simulink model "dwa"  (R2016a)
settings: Solver=VariableStepAuto  StartTime=0.0  StopTime=1  FixedStep=5e-5  RelTol=1e-3
values from neighbouring files (symbols this model uses):
  A_lpf = [-284 -370; 370 0]    [main.m]
  alpha = 0.5    [main.m]
  B_lpf = [440; 0]    [main.m]
  c = 3.5e-2    (= 0.035)    [main.m]
  C_lpf = [0 0.596]    [main.m]
  F_max = 250    [main.m]
  k = 42    [main.m]    (also in test_usw.m = [3,0.1])
  k_ac = 51    [main.m]
  k_af = 2.59e-2    (= 0.0259)    [main.m]
  L = 0.1    [main.m]
  m_c = 8.5    [main.m]
  m_f = 0.7e-3    (= 0.0007)    [main.m]
  n = 1e-18    [main.m]
  q1 = 1.53e-6    (= 1.53e-06)    [main.m]
  q2 = 0.465    [main.m]
  S = [-1.7e6 2.28e4 225 1.91 2.71]    [main.m]
  T = 0.55    [main.m]
  T_s = 5    [main.m]
undefined symbols (not defined in the file or in its folder): Discrete, sigbuilder_block, Time
libraries: simulink x1, ctrlSharedLib x1
settings Model: Creator=chao  LastModifiedBy=chao
settings GRTTargetCC: GeneratePreprocessorConditionals=Use local settings

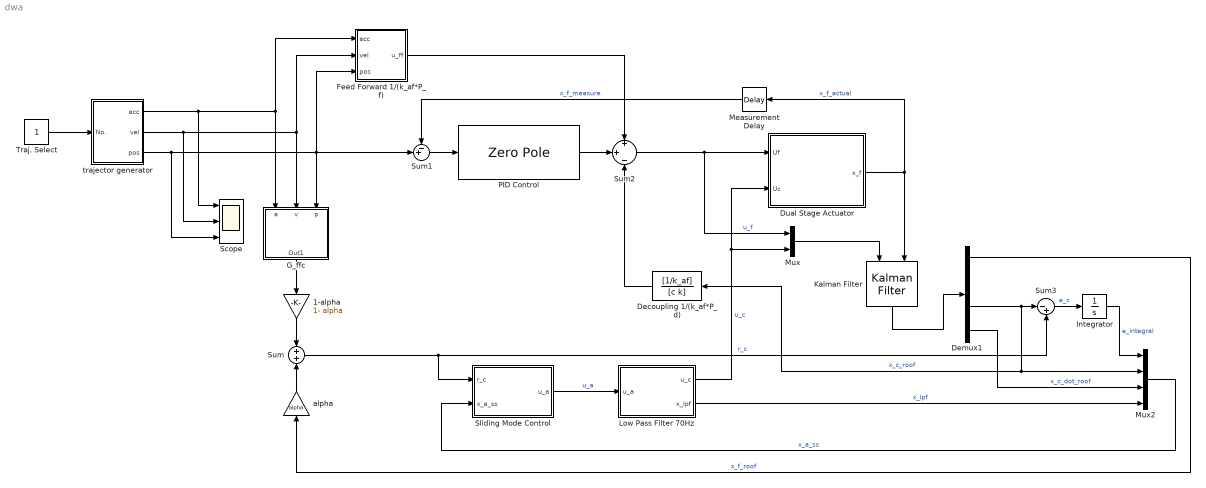
== system dwa ==
  1-alpha : Gain  Gain=1- alpha
  Decoupling 1/(k_af*P_d) : TransferFcn  Numerator=[1/k_af]  Denominator=[c k]
  Demux1 : Demux
  Dual Stage Actuator : Subsystem
  Feed Forward 1/(k_af*P_f) : Subsystem
  G_ffc : Subsystem
  Integrator : Integrator
  Kalman Filter : ctrlSharedLib/Kalman Filter  TimeDomain=Discrete-Time  UseCurrentEstimator=on  ModelSource=Individual A, B, C, D matrices  ModelSourceVariable=ss(0.95,1,1,0,1)  A=[0, 1, 0, 0; -k/m_f, -c/m_f, k/m_f, c/m_f;0, 0, 0, 1; 0, 0, 0, 0]  B=[0, 0; k_af/m_f, 0;0, 0; 0, k_ac/m_c];  C=[1 0 0 0]  D=[0 0]  NumberOfStates=1  NumberOfInputs=1  NumberOfOutputs=1  InitialEstimateSource=Dialog  X0=[0 0 0 0]  P0=10  UseK=off  UseGH=off  NumberOfProcessNoiseInputs=1  G=1  TimeInvariantG=on  H=0  TimeInvariantH=on  Q=[q1 0; 0 q2]  TimeInvariantQ=on  R=n  TimeInvariantR=on  N=0  TimeInvariantN=on  AddInputPort=on  AddEnablePort=off  OutputEstimatedY=off  OutputP=off  Ts=-1
  Low Pass Filter 70Hz : Subsystem
  Measurement Delay : TransportDelay  DelayTime=0
  Mux : Mux  Inputs=2
  Mux2 : Mux
  PID Control : ZeroPole  Zeros=[-2*pi*100 -2*pi*333]  Poles=[0 -2*pi*3000]  Gain=[3.2e6]
  Scope : Scope  NumInputPorts=3
  Sliding Mode Control : Subsystem
  Sum : Sum  Inputs=+|+
  Sum1 : Sum  Inputs=-+|
  Sum2 : Sum  Inputs=+|+|-
  Sum3 : Sum  Inputs=|-+
  Traj. Select : Constant
  alpha : Gain  Gain=alpha
  trajector generator : Subsystem
  wires:
  Sum1/1 -> PID Control/1
  PID Control/1 -> Sum2/2
  Sum2/1 -> Mux/1, Dual Stage Actuator/1(Uf)  "u_f"
  Feed Forward 1/(k_af*P_f)/1(u_ff) -> Sum2/1
  Measurement Delay/1 -> Sum1/1  "x_f_measure"
  Mux/1 -> Kalman Filter/1
  Sum3/1 -> Integrator/1  "e_c"
  Kalman Filter/1 -> Demux1/1
  Demux1/3 -> Mux2/2, Decoupling 1/(k_af*P_d)/1, Sum3/1  "x_c_roof"
  Dual Stage Actuator/1(x_f) -> Measurement Delay/1, Kalman Filter/2  "x_f_actual"
  Integrator/1 -> Mux2/1  "e_integral"
  Demux1/4 -> Mux2/3  "x_c_dot_roof"
  Low Pass Filter 70Hz/1(u_c) -> Dual Stage Actuator/2(Uc), Mux/2  "u_c"
  Mux2/1 -> Sliding Mode Control/2(x_a_ss)  "x_a_ss"
  Sliding Mode Control/1(u_a) -> Low Pass Filter 70Hz/1(u_a)  "u_a"
  Low Pass Filter 70Hz/2(x_lpf) -> Mux2/4  "x_lpf"
  Decoupling 1/(k_af*P_d)/1 -> Sum2/3
  alpha/1 -> Sum/2
  1-alpha/1 -> Sum/1
  Sum/1 -> Sliding Mode Control/1(r_c), Sum3/2  "r_c"
  Demux1/1 -> alpha/1  "x_f_roof"
  trajector generator/3(pos) -> Scope/3, Sum1/2, G_ffc/3(p), Feed Forward 1/(k_af*P_f)/3(pos)
  trajector generator/1(acc) -> Scope/1, G_ffc/1(a), Feed Forward 1/(k_af*P_f)/1(acc)
  trajector generator/2(vel) -> Scope/2, G_ffc/2(v), Feed Forward 1/(k_af*P_f)/2(vel)
  Traj. Select/1 -> trajector generator/1(No.)
  G_ffc/1(Out1) -> 1-alpha/1

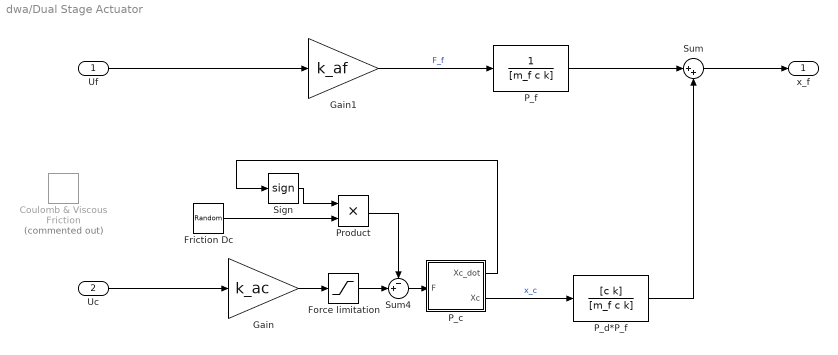
== system dwa/Dual Stage Actuator ==
  Uf : Inport
  Uc : Inport  Port=2
  Coulomb & Viscous Friction : simulink/Discontinuities/Coulomb & Viscous Friction  Commented=on  offset=[1 3 2 0]  gain=1
  Force limitation : Saturate  UpperLimit=F_max  LowerLimit=-F_max
  Friction Dc : RandomNumber  Mean=19  Variance=6.1^2  SampleTime=0.1
  Gain : Gain  Gain=k_ac
  Gain1 : Gain  Gain=k_af
  P_c : Subsystem
  P_d*P_f : TransferFcn  Numerator=[c k]  Denominator=[m_f c k]
  P_f : TransferFcn  Denominator=[m_f c k]
  Product : Product
  Sign : Signum
  Sum : Sum  Inputs=|++
  Sum4 : Sum  Inputs=-+|
  x_f : Outport
  wires:
  Gain1/1 -> P_f/1  "F_f"
  P_c/2(Xc) -> P_d*P_f/1  "x_c"
  Uf/1 -> Gain1/1
  Uc/1 -> Gain/1
  Gain/1 -> Force limitation/1
  Force limitation/1 -> Sum4/2
  Sum4/1 -> P_c/1(F)
  Friction Dc/1 -> Product/2
  Product/1 -> Sum4/1
  P_f/1 -> Sum/1
  Sum/1 -> x_f/1
  P_d*P_f/1 -> Sum/2
  P_c/1(Xc_dot) -> Sign/1
  Sign/1 -> Product/1

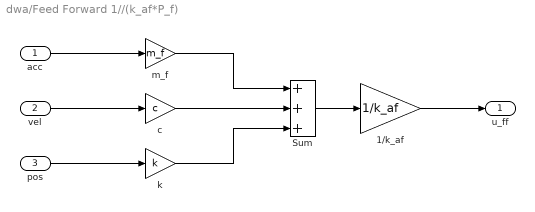
== system dwa/Feed Forward 1//(k_af*P_f) ==
  acc : Inport
  vel : Inport  Port=2
  pos : Inport  Port=3
  1/k_af : Gain  Gain=1/k_af
  Sum : Sum  Inputs=+++
  c : Gain  Gain=c
  k : Gain  Gain=k
  m_f : Gain  Gain=m_f
  u_ff : Outport
  wires:
  c/1 -> Sum/2
  acc/1 -> m_f/1
  pos/1 -> k/1
  k/1 -> Sum/3
  vel/1 -> c/1
  m_f/1 -> Sum/1
  1/k_af/1 -> u_ff/1
  Sum/1 -> 1/k_af/1

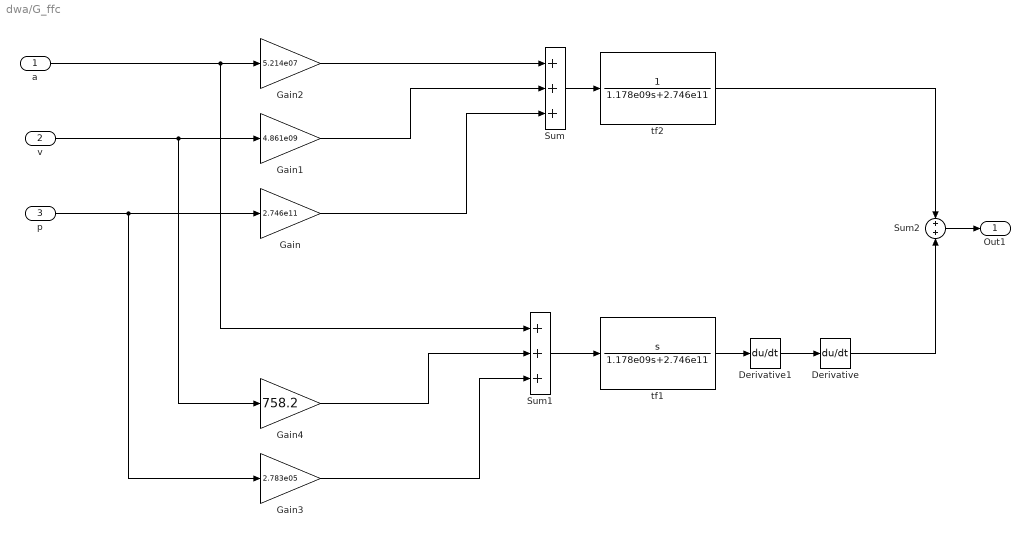
== system dwa/G_ffc ==
  a : Inport
  v : Inport  Port=2
  p : Inport  Port=3
  Derivative : Derivative
  Derivative1 : Derivative
  Gain : Gain  Gain=2.746e11
  Gain1 : Gain  Gain=4.861e09
  Gain2 : Gain  Gain=5.214e07
  Gain3 : Gain  Gain=2.783e05
  Gain4 : Gain  Gain=758.2
  Sum : Sum  Inputs=3
  Sum1 : Sum  Inputs=3
  Sum2 : Sum  Inputs=2
  tf1 : TransferFcn  Numerator="[1  0]"  Denominator=[1.178e09 2.746e11]
  tf2 : TransferFcn  Numerator=[1 ]  Denominator=[1.178e09 2.746e11]
  Out1 : Outport
  wires:
  Gain2/1 -> Sum/1
  Gain1/1 -> Sum/2
  Gain/1 -> Sum/3
  Derivative1/1 -> Derivative/1
  tf1/1 -> Derivative1/1
  p/1 -> Gain3/1, Gain/1
  v/1 -> Gain4/1, Gain1/1
  a/1 -> Sum1/1, Gain2/1
  Gain4/1 -> Sum1/2
  Gain3/1 -> Sum1/3
  Sum1/1 -> tf1/1
  Sum/1 -> tf2/1
  Sum2/1 -> Out1/1
  tf2/1 -> Sum2/1
  Derivative/1 -> Sum2/2

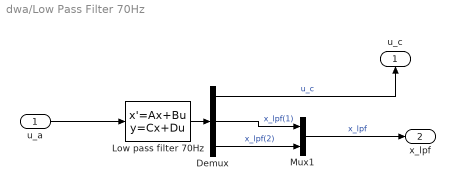
== system dwa/Low Pass Filter 70Hz ==
  u_a : Inport
  Demux : Demux  Outputs=3
  Low pass filter 70Hz : StateSpace  A=A_lpf  B=B_lpf  C=[C_lpf;1 0;0 1]  D=[0;0;0]  X0=0
  Mux1 : Mux  Description=x_lpf  Inputs=2
  u_c : Outport
  x_lpf : Outport  Port=2
  wires:
  Demux/3 -> Mux1/2  "x_lpf(2)"
  Demux/1 -> u_c/1  "u_c"
  Low pass filter 70Hz/1 -> Demux/1
  Mux1/1 -> x_lpf/1  "x_lpf"
  Demux/2 -> Mux1/1  "x_lpf(1)"
  u_a/1 -> Low pass filter 70Hz/1

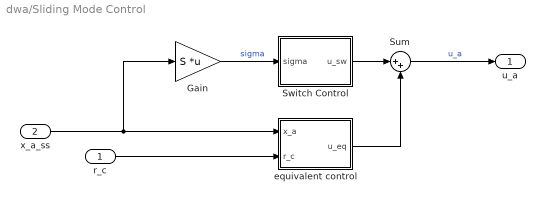
== system dwa/Sliding Mode Control ==
  r_c : Inport
  x_a_ss : Inport  Port=2
  Gain : Gain  Gain=S  Multiplication=Matrix(K*u)
  Sum : Sum  Inputs=|++
  Switch Control : MATLAB Function  TreatAsAtomicUnit=on
  equivalent control : MATLAB Function  TreatAsAtomicUnit=on
  u_a : Outport
  wires:
  r_c/1 -> equivalent control/2(r_c)
  Switch Control/1(u_sw) -> Sum/1
  equivalent control/1(u_eq) -> Sum/2
  Sum/1 -> u_a/1  "u_a"
  Gain/1 -> Switch Control/1(sigma)  "sigma"
  x_a_ss/1 -> equivalent control/1(x_a), Gain/1

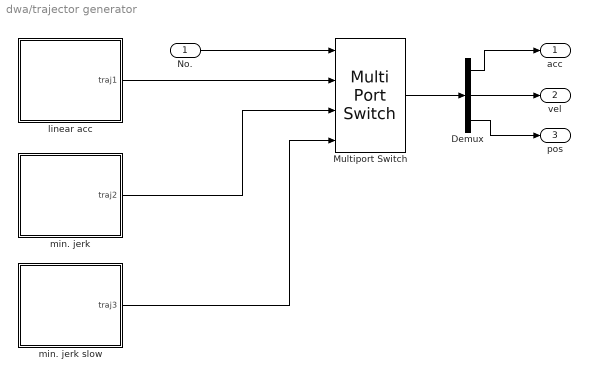
== system dwa/trajector generator ==
  No. : Inport
  Demux : Demux  Outputs=3
  Multiport Switch : MultiPortSwitch
  linear acc : Subsystem
  "min. jerk " : Subsystem
  min. jerk slow : Subsystem
  acc : Outport
  vel : Outport  Port=2
  pos : Outport  Port=3
  wires:
  Demux/1 -> acc/1
  Demux/2 -> vel/1
  Demux/3 -> pos/1
  Multiport Switch/1 -> Demux/1
  No./1 -> Multiport Switch/1
  linear acc/1(traj1) -> Multiport Switch/2
  "min. jerk "/1(traj2) -> Multiport Switch/3
  min. jerk slow/1(traj3) -> Multiport Switch/4

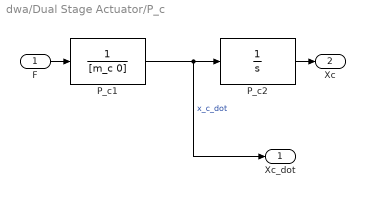
== system dwa/Dual Stage Actuator/P_c ==
  F : Inport
  P_c1 : TransferFcn  Denominator=[m_c 0]
  P_c2 : TransferFcn  Denominator=[1 0]
  Xc_dot : Outport
  Xc : Outport  Port=2
  wires:
  P_c2/1 -> Xc/1
  F/1 -> P_c1/1
  P_c1/1 -> Xc_dot/1, P_c2/1  "x_c_dot"

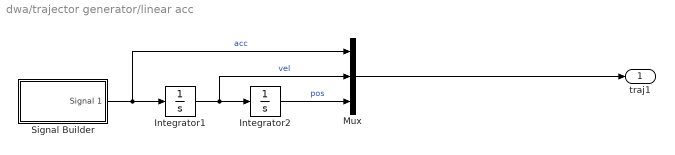
== system dwa/trajector generator/linear acc ==
  Integrator1 : Integrator
  Integrator2 : Integrator
  Mux : Mux  Inputs=3
  Signal Builder : Subsystem  Tag=STV Subsys  LoadFcn=sigbuilder_block('load');  StartFcn=sigbuilder_block('start');  StopFcn=sigbuilder_block('stop');  ClipboardFcn=sigbuilder_block('clipboard');  mask(Sigbuilder block){}
      mask help: Simulink:masks:SigbuilderBlock_MD
      mask init:
      | if ~strcmp(get_param(bdroot(gcbh),'SimulationStatus'),'stopped') tuvar = sigbuilder_block('maskInit'); end
      settings: CopyFcn=sigbuilder_block('copy');  DeleteFcn=sigbuilder_block('delete');  ModelCloseFcn=sigbuilder_block('modelClose');  PreSaveFcn=sigbuilder_block('preSave');  PauseFcn=sigbuilder_block('pause');  ContinueFcn=sigbuilder_block('continue');  NameChangeFcn=sigbuilder_block('namechange');  OpenFcn=sigbuilder_block('open',[436.2 135.6 550.8 400.2 ]);  CloseFcn=sigbuilder_block('close');
      mask Display: plot(0, 0, 100, 100,[2, 2, 32, 32, 2], [68, 8, 8, 68, 68],[32, 2], [38, 38], [32, 19, 2],[53, 60, 44], [32, 17, 17, 2],[16, 16, 31, 31]);txt = getActiveGroup(gcbh);text(2, 100, txt,'verticalAlignment', 'top');
  traj1 : Outport
  wires:
  Integrator1/1 -> Mux/2, Integrator2/1  "vel"
  Integrator2/1 -> Mux/3  "pos"
  Signal Builder/1(Signal 1) -> Mux/1, Integrator1/1  "acc"
  Mux/1 -> traj1/1

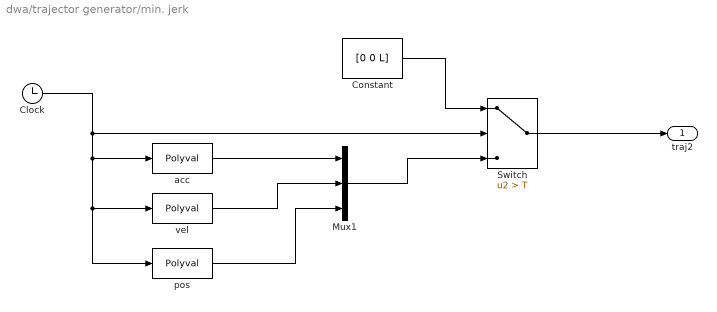
== system dwa/trajector generator/min. jerk  ==
  Clock : Clock
  Constant : Constant  Value=[0 0 L]
  Mux1 : Mux  Inputs=3
  Switch : Switch  Criteria=u2 > Threshold  Threshold=T
  acc : Polyval  Coefs=[120*L/(T^5), -180*L/(T^4), 60*L/(T^3), 0]
  pos : Polyval  Coefs=[6*L/(T^5), -15*L/(T^4), 10*L/(T^3), 0, 0, 0]
  vel : Polyval  Coefs=[30*L/(T^5), -60*L/(T^4), 30*L/(T^3), 0, 0]
  traj2 : Outport
  wires:
  Clock/1 -> pos/1, vel/1, acc/1, Switch/2
  Mux1/1 -> Switch/3
  Constant/1 -> Switch/1
  acc/1 -> Mux1/1
  pos/1 -> Mux1/3
  Switch/1 -> traj2/1
  vel/1 -> Mux1/2

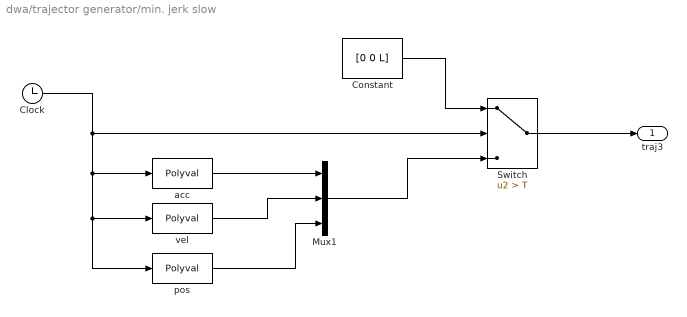
== system dwa/trajector generator/min. jerk slow ==
  Clock : Clock
  Constant : Constant  Value=[0 0 L]
  Mux1 : Mux  Inputs=3
  Switch : Switch  Criteria=u2 > Threshold  Threshold=T
  acc : Polyval  Coefs=[120*L/(T_s^5), -180*L/(T_s^4), 60*L/(T_s^3), 0]
  pos : Polyval  Coefs=[6*L/(T_s^5), -15*L/(T_s^4), 10*L/(T_s^3), 0, 0, 0]
  vel : Polyval  Coefs=[30*L/(T_s^5), -60*L/(T_s^4), 30*L/(T_s^3), 0, 0]
  traj3 : Outport
  wires:
  Clock/1 -> pos/1, vel/1, acc/1, Switch/2
  Mux1/1 -> Switch/3
  Constant/1 -> Switch/1
  acc/1 -> Mux1/1
  pos/1 -> Mux1/3
  Switch/1 -> traj3/1
  vel/1 -> Mux1/2

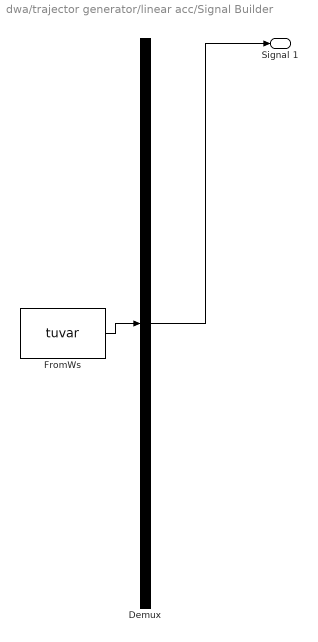
== system dwa/trajector generator/linear acc/Signal Builder ==
  Demux : Demux  Tag=STV Demux  Outputs=1
  FromWs : FromWorkspace  Tag=STV FromWs  VariableName=tuvar  SampleTime=0
      SigBuilderData=|
      | common.afterFinalStr = 'Extrapolate'
      | common.sampleTime = 0
      | dataSet.timeRange = [0 1]
      | dataSet.name = 'Group 1'
      | sbobj.Groups.Name = 'Group 1'
      | sbobj.Groups.Signals.Name = 'Signal 1'
      | sbobj.Groups.Signals.XData = [0 0.1 0.1 0.3 0.3 0.4 0.4 1]
      | sbobj.Groups.Signals.YData = [3.3 3.3 0 0 -3.3 -3.3 0 0]
      | sbobj.Groups.TimeRange = [0 1]
  Signal 1 : Outport  Tag=STV Outport
  wires:
  Demux/1 -> Signal 1/1
  FromWs/1 -> Demux/1

== matlab function dwa/Sliding Mode Control/Switch Control ==
  data: sigma input; u_sw output
function u_sw = fcn(sigma)
u_sw = (-k_sw1*sign(sigma)-k_sw2*sigma).*abs(2*sigmf(sigma,[k_sigm 0])-1);

== matlab function dwa/Sliding Mode Control/equivalent control ==
  data: x_a input; u_eq output; r_c input
function u_eq = fcn(x_a, r_c)
%#codegen
u_eq = -(S*B_au)\(S*A_a*x_a+S*B_ar*r_c);
